simulink model "ModelTest"  (R2019a)
settings: Solver=FixedStepDiscrete  StartTime=0.0  StopTime=10.0  FixedStep=0.1  RelTol=1e-3
libraries: simulink x4
settings Model: Creator=严龑  LastModifiedBy=严龑

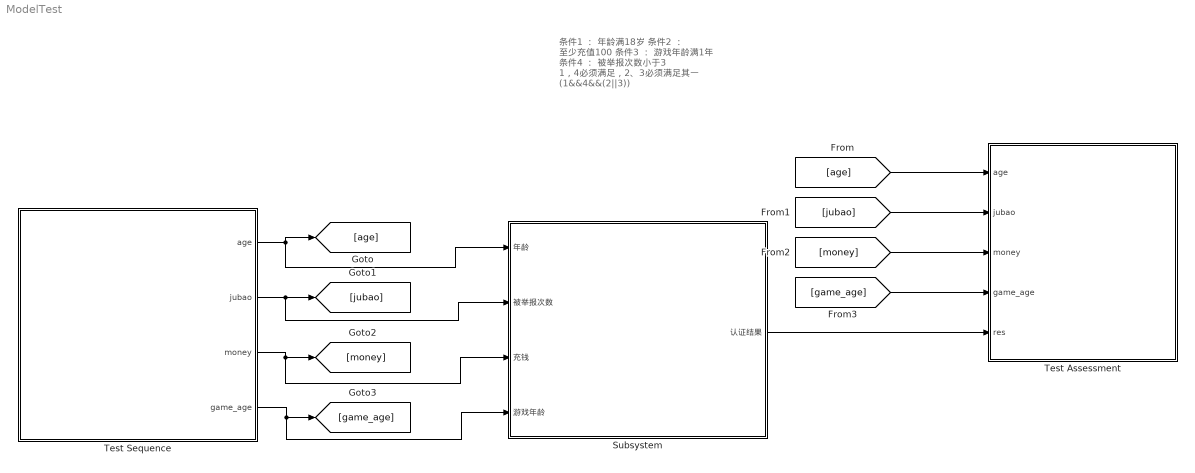
== system ModelTest ==
  note: 条件1 ： 年龄满18岁
      | 条件2 ： 至少充值100
      | 条件3 ： 游戏年龄满1年
      | 条件4 ： 被举报次数小于3
      | 1，4必须满足，2、3必须满足其一
      | (1&&4&&(2||3))
  Subsystem : Subsystem
  Test Assessment : Test Sequence  TreatAsAtomicUnit=on
  Test Sequence : Test Sequence  TreatAsAtomicUnit=on
  wires:
  Test Sequence/2(jubao) -> Subsystem/2(被举报次数), [jubao]
  Test Sequence/3(money) -> Subsystem/3(充钱), [money]
  Test Sequence/4(game_age) -> [game_age], Subsystem/4(游戏年龄)
  Test Sequence/1(age) -> [age], Subsystem/1(年龄)
  [age] -> Test Assessment/1(age)
  [jubao] -> Test Assessment/2(jubao)
  [money] -> Test Assessment/3(money)
  [game_age] -> Test Assessment/4(game_age)
  Subsystem/1(认证结果) -> Test Assessment/5(res)

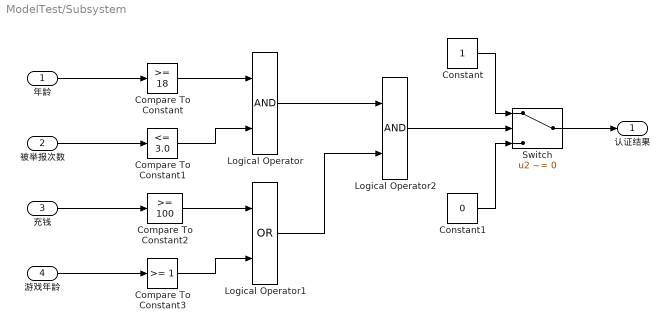
== system ModelTest/Subsystem ==
  年龄 : Inport
  被举报次数 : Inport  Port=2
  充钱 : Inport  Port=3
  游戏年龄 : Inport  Port=4
  Compare To Constant : simulink/Logic and Bit Operations/Compare To Constant  relop=>=  const=18  OutDataTypeStr=boolean
  Compare To Constant1 : simulink/Logic and Bit Operations/Compare To Constant  relop=<=  const=3.0  OutDataTypeStr=boolean
  Compare To Constant2 : simulink/Logic and Bit Operations/Compare To Constant  relop=>=  const=100  OutDataTypeStr=boolean
  Compare To Constant3 : simulink/Logic and Bit Operations/Compare To Constant  relop=>=  const=1  OutDataTypeStr=boolean
  Constant : Constant
  Constant1 : Constant  Value=0
  Logical Operator : Logic  AllPortsSameDT=off  OutDataTypeStr=boolean
  Logical Operator1 : Logic  Operator=OR  AllPortsSameDT=off  OutDataTypeStr=boolean
  Logical Operator2 : Logic  AllPortsSameDT=off  OutDataTypeStr=boolean
  Switch : Switch  Criteria=u2 ~= 0
  认证结果 : Outport
  wires:
  被举报次数/1 -> Compare To Constant1/1
  年龄/1 -> Compare To Constant/1
  充钱/1 -> Compare To Constant2/1
  游戏年龄/1 -> Compare To Constant3/1
  Compare To Constant/1 -> Logical Operator/1
  Compare To Constant1/1 -> Logical Operator/2
  Compare To Constant2/1 -> Logical Operator1/1
  Compare To Constant3/1 -> Logical Operator1/2
  Logical Operator/1 -> Logical Operator2/1
  Logical Operator1/1 -> Logical Operator2/2
  Logical Operator2/1 -> Switch/2
  Constant/1 -> Switch/1
  Constant1/1 -> Switch/3
  Switch/1 -> 认证结果/1

== stateflow chart ModelTest/Test Assessment ==
  settings: stateMachineType=SIMPLIFIED_MACHINE
  state Verification1
    state Successful
      verify(age>=18&&jubao<=3&&(money>=100||game_age>=1))
    state Verification1_1
    Verification1 -> (junction 22)
    (default) -> (junction 22)
    (junction 22) -> (junction 23) [order 1] : [res==1
        | ]
    (junction 23) -> Successful [order 1] : [~in(Successful)]
    (junction 23) -> (junction 26) [order 2]
    (junction 46) -> (junction 47)
    (junction 47) -> Verification1_1 [order 1] : [~in(Verification1_1)]
    (junction 47) -> (junction 50) [order 2]
    (junction 22) -> (junction 46) [order 2]
  (default) -> Verification1
  data: age input; jubao input; money input; game_age input; res input

== stateflow chart ModelTest/Test Sequence ==
  settings: stateMachineType=SIMPLIFIED_MACHINE
  state step_1
    age = 15
    money = 0
    game_age = 0.5
    jubao = 2
  state step_2
    age = 20
    money = 0
    game_age = 2
    jubao = 2
  state step_3
    age = 20
    money = 50
    game_age = 0.2
    jubao = 4
  (default) -> step_1
  step_1 -> step_2 : [
      | after(2,sec)
      | ]
  step_2 -> step_3 : [
      | after(3,sec)
      | ]
  data: age output; jubao output; money output; game_age output
